simulink model "Example_1_Closed"  (Simulink 8.3)
settings: Solver=ode45  StartTime=0.0  StopTime=40  RelTol=1e-3
libraries: simulink x1
settings Model: Creator=NeuControl  LastModifiedBy=Li Jinghao
settings DataIOCC: SignalLoggingSaveFormat=Dataset
settings DebuggingCC: UnderspecifiedInitializationDetection=Simplified  StateNameClashWarn=none
settings GRTTargetCC: CombineOutputUpdateFcns=on  GRTInterface=off

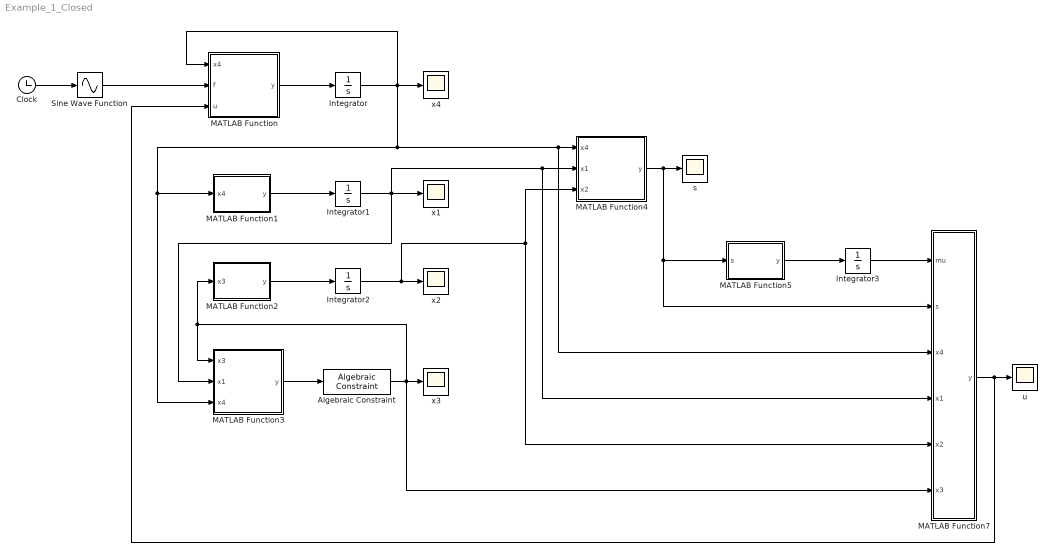
== system Example_1_Closed ==
  Algebraic Constraint : simulink/Math Operations/Algebraic Constraint  z0=0
  Clock : Clock
  Integrator : Integrator  InitialCondition=0.5*pi
  Integrator1 : Integrator  InitialCondition=0.3*pi
  Integrator2 : Integrator  InitialCondition=-5
  Integrator3 : Integrator
  MATLAB Function : MATLAB Function  TreatAsAtomicUnit=on
  MATLAB Function1 : MATLAB Function  TreatAsAtomicUnit=on
  MATLAB Function2 : MATLAB Function  TreatAsAtomicUnit=on
  MATLAB Function3 : MATLAB Function  TreatAsAtomicUnit=on
  MATLAB Function4 : MATLAB Function  TreatAsAtomicUnit=on
  MATLAB Function5 : MATLAB Function  TreatAsAtomicUnit=on
  MATLAB Function7 : MATLAB Function  TreatAsAtomicUnit=on
  Sine Wave Function : Sin  TimeSource=Use external signal  SampleTime=0
  s : Scope
      settings: SaveName=s
  u : Scope
      settings: SaveName=u
  x{1..4} (4 alike) : Scope
      x1 settings: SaveName=x1
      x2 settings: SaveName=x2
      x3 settings: SaveName=x3
      x4 settings: SaveName=x4
  wires:
  Clock/1 -> Sine Wave Function/1
  MATLAB Function/1(y) -> Integrator/1
  Integrator/1 -> MATLAB Function3/3(x4), MATLAB Function1/1(x4), MATLAB Function7/3(x4), MATLAB Function4/1(x4), MATLAB Function/1(x4), x4/1
  Sine Wave Function/1 -> MATLAB Function/2(f)
  MATLAB Function1/1(y) -> Integrator1/1
  Integrator1/1 -> MATLAB Function4/2(x1), MATLAB Function7/4(x1), MATLAB Function3/2(x1), x1/1
  MATLAB Function2/1(y) -> Integrator2/1
  Integrator2/1 -> MATLAB Function7/5(x2), MATLAB Function4/3(x2), x2/1
  Algebraic Constraint/1 -> MATLAB Function3/1(x3), MATLAB Function2/1(x3), MATLAB Function7/6(x3), x3/1
  MATLAB Function3/1(y) -> Algebraic Constraint/1
  MATLAB Function4/1(y) -> MATLAB Function7/2(s), MATLAB Function5/1(s), s/1
  MATLAB Function5/1(y) -> Integrator3/1
  Integrator3/1 -> MATLAB Function7/1(mu)
  MATLAB Function7/1(y) -> MATLAB Function/3(u), u/1

== matlab function MATLAB Function1 ==
  data: x4 input double; y output double
function y = fcn(x4)
%#codegen

Ll=5.5;
v=-1;
bt=2;
t0=0.5;

y = (v*bt/(Ll*t0))*x4;

== matlab function MATLAB Function ==
  data: x4 input double; f input double; u input double; y output double
function y = fcn(x4,f,u)
%#codegen

l=2.8;
Ll=5.5;
v=-1;
bt=2;
t0=0.5;

y = -v*bt/(Ll*t0)*x4+v*bt/(l*t0)*(u+f);

== matlab function MATLAB Function2 ==
  data: x3 input double; y output double
function y = fcn(x3)
%#codegen

v=-1;
bt=2;
t0=0.5;

y = (v*bt/t0)*x3;

== matlab function MATLAB Function3 ==
  data: x3 input double; x1 input double; x4 input double; y output double
function y = fcn(x3,x1,x4)
%#codegen

Ll=5.5;
v=-1;
bt=2;

y = sin(x1+(v*bt/(2*Ll))*x4)-x3;

== matlab function MATLAB Function4 ==
  data: x4 input double; x1 input double; x2 input double; y output double
function y = fcn(x4,x1,x2)
%#codegen

y = -1.5923*x1+5.4608*x2+x4;

== matlab function MATLAB Function5 ==
  data: s input double; y output double
function y = fcn(s)
%#codegen

delta=2;
beta=20;
epsilon=0.5;
l=2.8;
v=-1;
bt=2;
t0=0.5;
B1=v*bt/(l*t0);
bdf=1;
rho=norm(B1)*bdf;
k1=delta+1/beta*(rho*rho/(4*epsilon)+2*epsilon*rho+epsilon+2*epsilon*beta+8*epsilon^3);
k2=beta+4*epsilon^2+2*epsilon*k1;
k3=0.001;

y = -k2*(1/2*s/norm(s)+3/2*k3*s/sqrt(norm(s))+k3^2*s);

== matlab function MATLAB Function7 ==
  data: mu input double; s input double; x4 input double; y output double; x1 input double; x2 input double; x3 input double
function y = fcn(mu,s,x4,x1,x2,x3)
%#codegen

l=2.8;
Ll=5.5;
v=-1;
bt=2;
t0=0.5;
kappa=0.01;
xi=pi/2;
a=sin(xi)/xi;
x=[x1;x2;x3;x4];
v1=(sin(x1+v*bt/(2*Ll)*x4)-a)/(1-a);
v2=(1-sin(x1+v*bt/(2*Ll)*x4))/(1-a);

S=[-1.5923 5.4608 0 1];
E=[1 0 0 0;...
   0 1 0 0;...
   0 0 0 0;...
   0 0 0 1];
A1=[0 0     0    v*bt/(Ll*t0);...
    0 0 v*bt/t0       0;...
    1 0    -1    v*bt/(2*Ll);...
    0 0    0     -v*bt/(Ll*t0)];
A2=[0 0    0     v*bt/(Ll*t0);...
    0 0 v*bt/t0       0;...
    a 0   -1     a*v*bt/(2*Ll);...
    0 0   0      -v*bt/(Ll*t0)];
B1=v*bt/(l*t0);

delta=2;
beta=20;
epsilon=0.5;
bdf=1;
rho=norm(B1)*bdf;
k1=delta+1/beta*(rho*rho/(4*epsilon)+2*epsilon*rho+epsilon+2*epsilon*beta+8*epsilon^3);
k2=beta+4*epsilon^2+2*epsilon*k1;
k3=0.001;

y =-inv(B1)*(S*(v1*A1+v2*A2)*x+kappa*S*E*x+k1*(s/sqrt(norm(s))+k3*s)-mu);
